simulink model "tvr_sim"  (R2025b)
settings: Solver=ode4  StartTime=0.0  StopTime=120  RelTol=1e-3
values from neighbouring files (symbols this model uses):
  p = params()    [init_stabilizer_bode.m]    (also in loop_margin.m = setfield(p, f{:}, varargin{k+1}); setup.m)
libraries: simulink x2
settings Model: Creator=C4gie  LastModifiedBy=C4gie

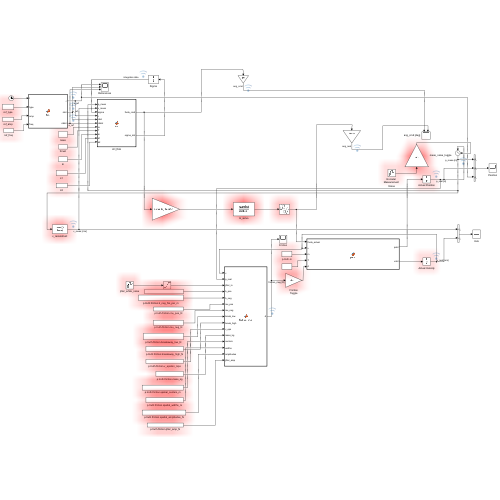
[thumbnail: Simulink's stored preview of the top-level diagram]
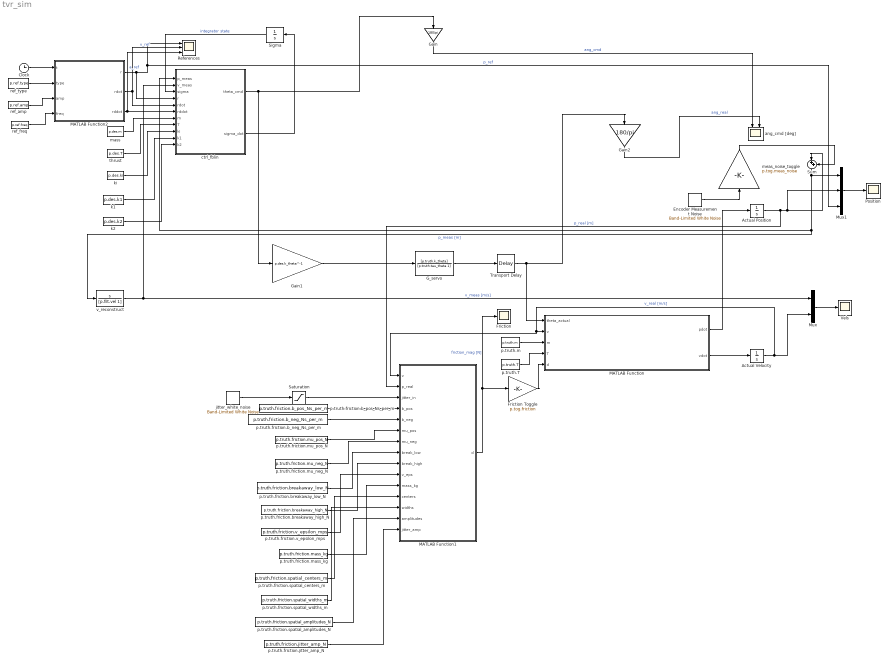
== system tvr_sim ==
  Actual Position : Integrator  InitialCondition=p.ic.p
  Actual Velocity : Integrator  InitialCondition=p.ic.v
  Clock : Clock
  Encoder Measurement Noise : simulink/Sources/Band-Limited White Noise  Cov=1e-09  Ts=0.001  seed=[p.seed.meas]
  Friction : Scope
      settings: ActiveDisplayYMinimum=-3.4761991078381564  ActiveDisplayYMaximum=3.1351501426415305  DataLoggingVariableName=ScopeData3
  Friction Toggle : Gain  Gain=p.tog.friction
  G_servo : TransferFcn  Numerator=[p.truth.k_theta]  Denominator=[p.truth.tau_theta 1]
  Gain : Gain  Gain=180/pi
  Gain1 : Gain  Gain=p.des.k_theta^-1
  Gain2 : Gain  Gain=180/pi
  MATLAB Function : MATLAB Function  TreatAsAtomicUnit=on
  MATLAB Function1 : MATLAB Function  TreatAsAtomicUnit=on
  MATLAB Function2 : MATLAB Function  TreatAsAtomicUnit=on
  Mux : Mux  Inputs=2
      settings: DisplayOption=signals
  Mux1 : Mux  Inputs=3
      settings: DisplayOption=signals
  Position : Scope
      settings: ActiveDisplayYMinimum=-0.053672788114687793  ActiveDisplayYMaximum=0.0615373322216633
  References : Scope  NumInputPorts=3
      settings: ActiveDisplayYMinimum=-0.77017009761882271  ActiveDisplayYMaximum=0.64793197793962221  DataLoggingVariableName=ScopeData2
  Saturation : Saturate  UpperLimit=1  LowerLimit=-1
  Sigma : Integrator
  Sum : Sum  Inputs=|++
  Transport Delay : TransportDelay  DelayTime=p.truth.L_theta  PadeOrder=3
  Vels : Scope
      settings: ActiveDisplayYMinimum=-0.25240521521328124  ActiveDisplayYMaximum=0.30674414454184945  DataLoggingVariableName=ScopeData4
  ang_cmd [deg] : Scope  NumInputPorts=2
      settings: ActiveDisplayYMinimum=-64.262247595653918  ActiveDisplayYMaximum=67.567814662811415
  ctrl_fblin : MATLAB Function  TreatAsAtomicUnit=on
  jitter_white_noise : simulink/Sources/Band-Limited White Noise  Cov=[0.01]  Ts=0.1  seed=[p.seed.friction]
  k1 : Constant  Value=p.des.k1
  k2 : Constant  Value=p.des.k2
  ki : Constant  Value=p.des.ki
  mass : Constant  Value=p.des.m
  meas_noise_toggle : Gain  Gain=p.tog.meas_noise
  p.truth.T : Constant  Value=p.truth.T
  p.truth.friction.b_neg_Ns_per_m : Constant  Value=p.truth.friction.b_neg_Ns_per_m
  p.truth.friction.b_pos_Ns_per_m : Constant  Value=p.truth.friction.b_pos_Ns_per_m
  p.truth.friction.breakaway_high_N : Constant  Value=p.truth.friction.breakaway_high_N
  p.truth.friction.breakaway_low_N : Constant  Value=p.truth.friction.breakaway_low_N
  p.truth.friction.jitter_amp_N : Constant  Value=p.truth.friction.jitter_amp_N
  p.truth.friction.mass_kg : Constant  Value=p.truth.friction.mass_kg
  p.truth.friction.mu_neg_N : Constant  Value=p.truth.friction.mu_neg_N
  p.truth.friction.mu_pos_N : Constant  Value=p.truth.friction.mu_pos_N
  p.truth.friction.spatial_amplitudes_N : Constant  Value=p.truth.friction.spatial_amplitudes_N
  p.truth.friction.spatial_centers_m : Constant  Value=p.truth.friction.spatial_centers_m
  p.truth.friction.spatial_widths_m : Constant  Value=p.truth.friction.spatial_widths_m
  p.truth.friction.v_epsilon_mps : Constant  Value=p.truth.friction.v_epsilon_mps
  p.truth.m : Constant  Value=p.truth.m
  ref_amp : Constant  Value=p.ref.amp
  ref_freq : Constant  Value=p.ref.freq
  ref_type : Constant  Value=p.ref.type
  thrust : Constant  Value=p.des.T
  v_reconstruct : TransferFcn  Numerator=[1 0]  Denominator=[p.filt.vel 1]
  wires:
  Clock/1 -> MATLAB Function2/1(t)
  p.truth.friction.spatial_widths_m/1 -> MATLAB Function1/13(widths)
  p.truth.friction.mu_neg_N/1 -> MATLAB Function1/7(mu_neg)
  ref_freq/1 -> MATLAB Function2/4(freq)
  MATLAB Function2/3(rddot) -> ctrl_fblin/6(rddot), References/3  "a_ref"
  p.truth.friction.spatial_centers_m/1 -> MATLAB Function1/12(centers)
  p.truth.friction.mass_kg/1 -> MATLAB Function1/11(mass_kg)
  MATLAB Function2/2(rdot) -> References/2, ctrl_fblin/5(rdot)  "v_ref"
  p.truth.m/1 -> MATLAB Function/3(m)
  p.truth.friction.jitter_amp_N/1 -> MATLAB Function1/15(jitter_amp)
  p.truth.friction.spatial_amplitudes_N/1 -> MATLAB Function1/14(amplitudes)
  MATLAB Function2/1(r) -> Mux1/3, References/1, ctrl_fblin/4(r)  "p_ref"
  p.truth.friction.v_epsilon_mps/1 -> MATLAB Function1/10(v_eps)
  p.truth.friction.breakaway_low_N/1 -> MATLAB Function1/8(break_low)
  p.truth.friction.mu_pos_N/1 -> MATLAB Function1/6(mu_pos)
  ref_type/1 -> MATLAB Function2/2(type)
  jitter_white_noise/1 -> Saturation/1
  mass/1 -> ctrl_fblin/7(m)
  ki/1 -> ctrl_fblin/9(ki)
  ref_amp/1 -> MATLAB Function2/3(amp)
  G_servo/1 -> Transport Delay/1
  Sigma/1 -> ctrl_fblin/3(sigma)  "integrator state"
  thrust/1 -> ctrl_fblin/8(T)
  k1/1 -> ctrl_fblin/10(k1)
  k2/1 -> ctrl_fblin/11(k2)
  Mux/1 -> Vels/1
  v_reconstruct/1 -> Mux/1, ctrl_fblin/2(v_meas)  "v_meas [m/s]"
  ctrl_fblin/1(theta_cmd) -> Gain/1, Gain1/1
  ctrl_fblin/2(sigma_dot) -> Sigma/1
  Gain1/1 -> G_servo/1
  Mux1/1 -> Position/1
  Saturation/1 -> MATLAB Function1/3(jitter_in)
  p.truth.friction.b_pos_Ns_per_m/1 -> MATLAB Function1/4(b_pos)
  p.truth.friction.b_neg_Ns_per_m/1 -> MATLAB Function1/5(b_neg)
  meas_noise_toggle/1 -> Sum/2
  p.truth.friction.breakaway_high_N/1 -> MATLAB Function1/9(break_high)
  Gain/1 -> ang_cmd [deg]/1  "ang_cmd"
  MATLAB Function1/1(d) -> Friction/1, Friction Toggle/1  "friction_mag [N]"
  Transport Delay/1 -> Gain2/1, MATLAB Function/1(theta_actual)
  p.truth.T/1 -> MATLAB Function/4(T)
  Friction Toggle/1 -> MATLAB Function/5(d)
  Gain2/1 -> ang_cmd [deg]/2  "ang_real"
  Encoder Measurement Noise/1 -> meas_noise_toggle/1
  MATLAB Function/1(pdot) -> Actual Position/1
  MATLAB Function/2(vdot) -> Actual Velocity/1
  Actual Position/1 -> Sum/1, Mux1/2, MATLAB Function1/2(p_real)  "p_real [m]"
  Sum/1 -> v_reconstruct/1, ctrl_fblin/1(p_meas), Mux1/1  "p_meas [m]"
  Actual Velocity/1 -> MATLAB Function1/1(v), MATLAB Function/2(v), Mux/2  "v_real [m/s]"

== matlab function tvr_sim/MATLAB Function1 ==
  data: v input; p_real input; jitter_in input; b_pos input; d output; b_neg input; mu_pos input; mu_neg input; break_low input; break_high input; v_eps input; mass_kg input; centers input; widths input; amplitudes input; jitter_amp input
function d = friction_mc(v, p_real, jitter_in, b_pos, b_neg, mu_pos, mu_neg, break_low, break_high, v_eps, mass_kg, centers, widths, amplitudes, jitter_amp)
  d = friction_mc_fields(v, p_real, jitter_in, b_pos, b_neg, mu_pos, mu_neg, break_low, break_high, v_eps, mass_kg, centers, widths, amplitudes, jitter_amp);
end

== matlab function tvr_sim/ctrl_fblin ==
  data: p_meas input; theta_cmd output; v_meas input; sigma input; r input; rdot input; rddot input; m input; T input; ki input; k1 input; k2 input; sigma_dot output
function [theta_cmd, sigma_dot] = fcn(p_meas, v_meas, sigma, r, rdot, rddot, m, T, ki, k1, k2)
  [theta_cmd, sigma_dot] = ctrl_fblin(p_meas, v_meas, sigma, r, rdot, rddot, m, T, ki, k1, k2);
end

== matlab function tvr_sim/MATLAB Function ==
  data: theta_actual input; pdot output; v input; m input; T input; d input; vdot output
function [pdot, vdot] = plant(theta_actual, v, m, T, d)
  [pdot, vdot] = plant(theta_actual, v, m, T, d);
end

== matlab function tvr_sim/MATLAB Function2 ==
  data: t input; r output; type input; amp input; freq input; rdot output; rddot output
function [r, rdot, rddot] = fcn(t, type, amp, freq)
    [r, rdot, rddot] = ref_gen(t, type, amp, freq);
end
